simulink library "Library"  (R2020b)
settings: Solver=VariableStepAuto  StartTime=0.0  StopTime=10.0  RelTol=1e-3
undefined symbols (not defined in the file or in its folder): DiscIntNeverNeededParam
libraries: simulink x1
settings Model: Creator=elbit  LastModifiedBy=elbit

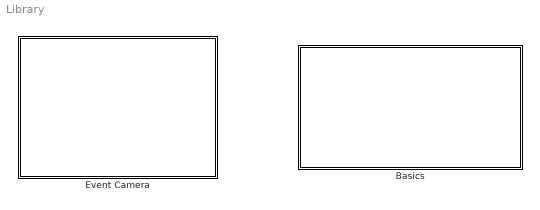
== system Library ==
  Basics : Subsystem
  Event Camera : Subsystem

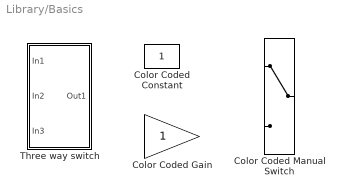
== system Library/Basics ==
  Color Coded Constant : Constant  OutDataTypeStr=boolean
      settings: OpenFcn=|
      | if get_param(gcbh,'value')-48 set_param(gcbh,'value','0','backgroundcolor','red');
      | else set_param(gcbh,'value','1','backgroundcolor','green');
      | end
  Color Coded Manual Switch : ManualSwitch
      settings: OpenFcn=|
      | sw = get_param(gcb,'sw');
      | if strcmp(sw,'1')
      | set_param(gcb,'sw','0');
      | else
      | set_param(gcb,'sw','1');
      | end
      | if strcmp(sw,'1')
      |     set_param(gcb,'backgroundcolor','red')
      | else
      |     set_param(gcb,'backgroundcolor','green')
      | end
  Color Coded Gain : Gain  OutDataTypeStr=Inherit: Same as input
      settings: OpenFcn=|
      | if get_param(gcbh,'gain')-48 set_param(gcbh,'gain','0','backgroundcolor','red');
      | else set_param(gcbh,'gain','1','backgroundcolor','green');
      | end
  Three way switch : Subsystem  mask{Choice=1}
      mask prompts: Choice "Numer of port to output"
      settings: OpenFcn=|
      | Choice=get_param(gcbh,'Choice');
      | Choice=str2num(Choice)+1;
      | if Choice==4, Choice=1; end
      | set_param(gcbh,'Choice',num2str(Choice));
      mask Display:
      | %plot box
      | plot([-1,1,1,-1],[-1,-1,1,1]);
      | 
      | %plot circles
      | t=linspace(0,2*pi,20);
      | r=0.1;
      | x=r*cos(t); y=0.4*r*sin(t);
      | plot(x-0.9,y+0.7);
      | plot(x-0.9,y);
      | plot(x-0.9,y-0.7);
      | 
      | %plot line
      | switch Choice
      |     case 1
      |         plot([-0.8,0,1],0.7*[1,0,0]);
      |     case 2
      |         plot([-0.8,0,1],[0,0,0]);
      |     case 3
      |         plot([-0.8,0,1],0.7*[-1,0,0]);
      | end

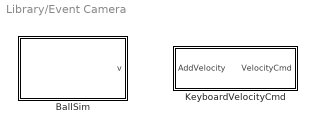
== system Library/Event Camera ==
  BallSim : Subsystem  mask{vlim=deg2rad(10)*[0,1], xlim=deg2rad(10)*[0,1], Tswitch=3}
      mask prompts: vlim "abs vlim range"; xlim "xlim range"
  KeyboardVelocityCmd : Subsystem  mask{max=20*pi/180, step_percentile=0.2}

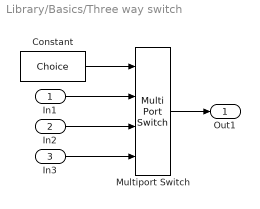
== system Library/Basics/Three way switch ==
  In1 : Inport
  In2 : Inport  Port=2
  In3 : Inport  Port=3
  Constant : Constant  Value=Choice
  Multiport Switch : MultiPortSwitch
  Out1 : Outport
  wires:
  Constant/1 -> Multiport Switch/1
  In3/1 -> Multiport Switch/4
  In2/1 -> Multiport Switch/3
  Multiport Switch/1 -> Out1/1
  In1/1 -> Multiport Switch/2

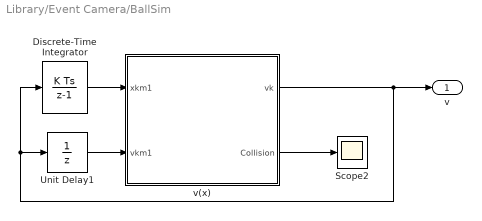
== system Library/Event Camera/BallSim ==
  Discrete-Time Integrator : DiscreteIntegrator  SampleTime=-1  ICPrevOutput=DiscIntNeverNeededParam  ICPrevScaledInput=DiscIntNeverNeededParam
  Scope2 : Scope
  Unit Delay1 : UnitDelay  SampleTime=-1  HasFrameUpgradeWarning=on
  v(x) : Stateflow chart  TreatAsAtomicUnit=on
  v : Outport
  wires:
  v(x)/1(vk) -> v/1, Discrete-Time Integrator/1, Unit Delay1/1
  v(x)/2(Collision) -> Scope2/1
  Discrete-Time Integrator/1 -> v(x)/1(xkm1)
  Unit Delay1/1 -> v(x)/2(vkm1)

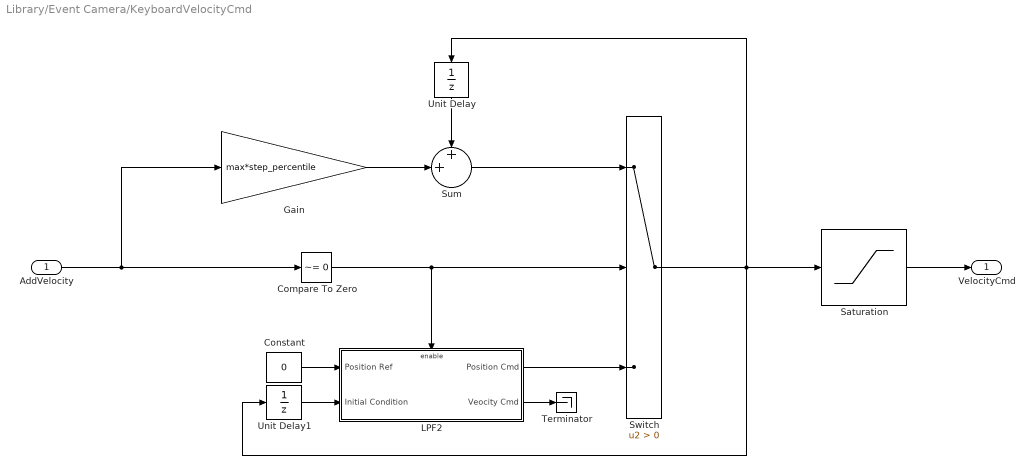
== system Library/Event Camera/KeyboardVelocityCmd ==
  AddVelocity : Inport
  Compare To Zero : simulink/Logic and Bit Operations/Compare To Zero  relop=~=  OutDataTypeStr=boolean
  Constant : Constant  Value=0  OutDataTypeStr=Inherit: Inherit via back propagation
  Gain : Gain  Gain=max*step_percentile
  LPF2 : Subsystem  mask{PosBW=1, Vel_Max=inf, Vel_Min=-inf}
      mask prompts: PosBW "Position BW [Hz]"; Vel_Max "Maximum Velocity"; Vel_Min "Minimum Velocity"
      mask Display: fprintf('Resetable LPF %.3g[Hz] \n/w Vel Limits',PosBW);
  Saturation : Saturate  UpperLimit=max  LowerLimit=-max
  Sum : Sum  Inputs=++|
  Switch : Switch  Criteria=u2 > Threshold
  Terminator : Terminator
  Unit Delay : UnitDelay  SampleTime=-1  HasFrameUpgradeWarning=on
  Unit Delay1 : UnitDelay  SampleTime=-1  HasFrameUpgradeWarning=on
  VelocityCmd : Outport
  wires:
  Saturation/1 -> VelocityCmd/1
  Unit Delay1/1 -> LPF2/2(Initial Condition)
  Constant/1 -> LPF2/1(Position Ref)
  AddVelocity/1 -> Gain/1, Compare To Zero/1
  Compare To Zero/1 -> Switch/2, LPF2/Enable
  LPF2/2(Veocity Cmd) -> Terminator/1
  LPF2/1(Position Cmd) -> Switch/3
  Switch/1 -> Saturation/1, Unit Delay/1, Unit Delay1/1
  Unit Delay/1 -> Sum/1
  Gain/1 -> Sum/2
  Sum/1 -> Switch/1

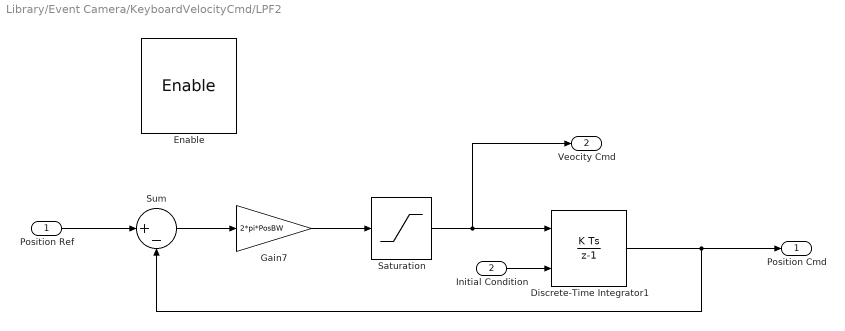
== system Library/Event Camera/KeyboardVelocityCmd/LPF2 ==
  Position Ref : Inport
  Initial Condition : Inport  Port=2
  Enable : EnablePort  StatesWhenEnabling=reset
  Discrete-Time Integrator1 : DiscreteIntegrator  InitialConditionSource=external  SampleTime=-1  ICPrevOutput=DiscIntNeverNeededParam  ICPrevScaledInput=DiscIntNeverNeededParam
  Gain7 : Gain  Gain=2*pi*PosBW
  Saturation : Saturate  UpperLimit=Vel_Max  LowerLimit=Vel_Min
  Sum : Sum  Inputs=|+-
  Position Cmd : Outport  VectorParamsAs1DForOutWhenUnconnected=off
  Veocity Cmd : Outport  Port=2  VectorParamsAs1DForOutWhenUnconnected=off
  wires:
  Initial Condition/1 -> Discrete-Time Integrator1/2
  Saturation/1 -> Discrete-Time Integrator1/1, Veocity Cmd/1
  Discrete-Time Integrator1/1 -> Sum/2, Position Cmd/1
  Gain7/1 -> Saturation/1
  Sum/1 -> Gain7/1
  Position Ref/1 -> Sum/1

== stateflow chart Library/Event Camera/BallSim/v(x) ==
  state Moving
    during:
    vk=vkm1;
    Collision=false;
  state OnEdge
    entry:
    normal=ComputeNormal(xkm1);
    if (vkm1'*normal)<0
    Collision=true;
    vk=UpdateV(vkm1,normal);
    end
  Moving -> OnEdge : [QOnEdge(xkm1) || after(Tswitch,'sec')]
  (default) -> Moving
  (junction 53) -> Moving
  OnEdge -> (junction 51)
  (junction 51) -> (junction 53)
  data: x function_input; Q function_output; v_in function_input; n function_input; v_out function_output; x function_input; n function_output; vk output =(vlim(1)+diff(vlim)*rand)*randSign(); normal local; xkm1 input; vkm1 input; xlim parameter; vlim parameter; Collision output; Tswitch parameter
  function Q=QOnEdge(x):
    | function Q=QOnEdge(x)
    | 
    | if x(1)>xlim(1) && x(1)<xlim(2)
    |     Q=false;
    | else
    |     Q=true;
    | end
  function v_out=UpdateV(v_in,n):
    | function v_out=UpdateV(v_in,n)
    | %written for N dimensions, but used with one
    | v_mirror=v_in-2*(v_in'*n)*n;
    | vabs=abs(vlim(1)+diff(vlim)*rand);% max(rand*vlim(2),vlim(1));
    | v_out = v_mirror/vecnorm(v_mirror)*vabs;
    | end
  function n=ComputeNormal(x):
    | function n=ComputeNormal(x)
    | %xlim - [xmin,xmax];
    | [~,ind]=min(abs(([x,x]-xlim)'));
    | if ind==1
    |         n=1;
    | else
    |         n=-1;
    | end
